simulink library "MBDS_Subsystems"  (R2018b)
settings: Solver=ode45  StartTime=0.0  StopTime=10.0  RelTol=1e-3
libraries: KIBES_Signal x1429, MBDS_Modules x44, simulink x2
(part 10 of 15)

== system MBDS_Subsystems/SUB_IoControl/AnalogsSupply ==
  bo_SendEnable : Inport
  AND : Subsystem  InitFcn=|  mask(AND){MBDS_LibraryBlock=on, BitwiseMode=off, Inputs=2, UseBitMask=off, BitMask='A7', OutDataTypeStr=Inherit: Inherit via back propagation, MBDS_BlockVersion=08.20.02}
      | if(exist('MBDS_BlockCallback', 'file'))
      |    MBDS_BlockCallback('Update', gcb);
      | end
      mask prompts: MBDS_LibraryBlock "MBDS library block"; BitwiseMode "Use 'bitwise' mode"; Inputs "Number of input ports:"; UseBitMask "Use bit mask"; BitMask "Bit mask:"; OutDataTypeStr "Output data type:"; MBDS_BlockVersion "Version:"
      mask help: Logical or bitwise AND operator. For multiple inputs, operators are applied across the inputs. For a single input, operators are applied across the input vector. In bitwise mode a bit mask can be applied onto single input signals.
      mask init: same as MBDS_Subsystems/SUB_DateTime/AND
      mask Help: eval(['open([workdir(''library_dir:''),''\Blockset\help\'',get_param(gcb,''MaskType''),''.html''])'])
      mask Callback BitwiseMode:
      | if(exist('MBDS_BlockCallback', 'file'))
      |    MBDS_BlockCallback('BitwiseMode', gcb);
      | end
      mask Callback Inputs:
      | if(exist('MBDS_BlockCallback', 'file'))
      |    MBDS_BlockCallback('Inputs', gcb);
      | end
      mask Callback UseBitMask:
      | if(exist('MBDS_BlockCallback', 'file'))
      |    MBDS_BlockCallback('UseBitMask', gcb);
      | end
      mask Callback BitMask:
      | if(exist('MBDS_BlockCallback', 'file'))
      |    MBDS_BlockCallback('BitMask', gcb);
      | end
      mask TypeOptions OutDataTypeStr: Inherit: Inherit via back propagation | int8 | uint8 | int16 | uint16 | int32 | uint32 | boolean
      mask Callback OutDataTypeStr:
      | % Adopt Value
      | if(exist('MBDS_BlockCallback', 'file'))
      |    MBDS_BlockCallback('OutDataTypeStr', gcb);
      | end
      mask DialogControl ParameterTabVar0 Prompt: Main
      mask DialogControl ParameterTabVar01 Prompt: Signal Attributes
      mask DialogControl ParameterTabVar012 Prompt: Version
      mask Display:
      | % Show icon or block text
      | if(UseBitMask)
      |    if(isnumeric(BitMask))
      |       BitMaskString = ['0x',dec2hex(floor(BitMask))];
      |    elseif(ischar(BitMask))
      |       BitMaskString = ['0x',upper(BitMask)];
      |    else
      |       BitMaskString = '???';
      |    end
      |    disp(sprintf(['AND\n', BitMaskString]))
      | else
      |    disp('AND')
      | end
  AND1 : Subsystem  InitFcn=|  mask(AND){MBDS_LibraryBlock=on, BitwiseMode=off, Inputs=2, UseBitMask=off, BitMask='A7', OutDataTypeStr=Inherit: Inherit via back propagation, MBDS_BlockVersion=08.20.02}
      | if(exist('MBDS_BlockCallback', 'file'))
      |    MBDS_BlockCallback('Update', gcb);
      | end
      mask prompts: MBDS_LibraryBlock "MBDS library block"; BitwiseMode "Use 'bitwise' mode"; Inputs "Number of input ports:"; UseBitMask "Use bit mask"; BitMask "Bit mask:"; OutDataTypeStr "Output data type:"; MBDS_BlockVersion "Version:"
      mask help: Logical or bitwise AND operator. For multiple inputs, operators are applied across the inputs. For a single input, operators are applied across the input vector. In bitwise mode a bit mask can be applied onto single input signals.
      mask init: same as MBDS_Subsystems/SUB_DateTime/AND
      mask Help: eval(['open([workdir(''library_dir:''),''\Blockset\help\'',get_param(gcb,''MaskType''),''.html''])'])
      mask Callback BitwiseMode:
      | if(exist('MBDS_BlockCallback', 'file'))
      |    MBDS_BlockCallback('BitwiseMode', gcb);
      | end
      mask Callback Inputs:
      | if(exist('MBDS_BlockCallback', 'file'))
      |    MBDS_BlockCallback('Inputs', gcb);
      | end
      mask Callback UseBitMask:
      | if(exist('MBDS_BlockCallback', 'file'))
      |    MBDS_BlockCallback('UseBitMask', gcb);
      | end
      mask Callback BitMask:
      | if(exist('MBDS_BlockCallback', 'file'))
      |    MBDS_BlockCallback('BitMask', gcb);
      | end
      mask TypeOptions OutDataTypeStr: Inherit: Inherit via back propagation | int8 | uint8 | int16 | uint16 | int32 | uint32 | boolean
      mask Callback OutDataTypeStr:
      | % Adopt Value
      | if(exist('MBDS_BlockCallback', 'file'))
      |    MBDS_BlockCallback('OutDataTypeStr', gcb);
      | end
      mask DialogControl ParameterTabVar0 Prompt: Main
      mask DialogControl ParameterTabVar01 Prompt: Signal Attributes
      mask DialogControl ParameterTabVar012 Prompt: Version
      mask Display:
      | % Show icon or block text
      | if(UseBitMask)
      |    if(isnumeric(BitMask))
      |       BitMaskString = ['0x',dec2hex(floor(BitMask))];
      |    elseif(ischar(BitMask))
      |       BitMaskString = ['0x',upper(BitMask)];
      |    else
      |       BitMaskString = '???';
      |    end
      |    disp(sprintf(['AND\n', BitMaskString]))
      | else
      |    disp('AND')
      | end
  AND2 : Subsystem  InitFcn=|  mask(AND){MBDS_LibraryBlock=on, BitwiseMode=off, Inputs=2, UseBitMask=off, BitMask='A7', OutDataTypeStr=Inherit: Inherit via back propagation, MBDS_BlockVersion=08.20.02}
      | if(exist('MBDS_BlockCallback', 'file'))
      |    MBDS_BlockCallback('Update', gcb);
      | end
      mask prompts: MBDS_LibraryBlock "MBDS library block"; BitwiseMode "Use 'bitwise' mode"; Inputs "Number of input ports:"; UseBitMask "Use bit mask"; BitMask "Bit mask:"; OutDataTypeStr "Output data type:"; MBDS_BlockVersion "Version:"
      mask help: Logical or bitwise AND operator. For multiple inputs, operators are applied across the inputs. For a single input, operators are applied across the input vector. In bitwise mode a bit mask can be applied onto single input signals.
      mask init: same as MBDS_Subsystems/SUB_DateTime/AND
      mask Help: eval(['open([workdir(''library_dir:''),''\Blockset\help\'',get_param(gcb,''MaskType''),''.html''])'])
      mask Callback BitwiseMode:
      | if(exist('MBDS_BlockCallback', 'file'))
      |    MBDS_BlockCallback('BitwiseMode', gcb);
      | end
      mask Callback Inputs:
      | if(exist('MBDS_BlockCallback', 'file'))
      |    MBDS_BlockCallback('Inputs', gcb);
      | end
      mask Callback UseBitMask:
      | if(exist('MBDS_BlockCallback', 'file'))
      |    MBDS_BlockCallback('UseBitMask', gcb);
      | end
      mask Callback BitMask:
      | if(exist('MBDS_BlockCallback', 'file'))
      |    MBDS_BlockCallback('BitMask', gcb);
      | end
      mask TypeOptions OutDataTypeStr: Inherit: Inherit via back propagation | int8 | uint8 | int16 | uint16 | int32 | uint32 | boolean
      mask Callback OutDataTypeStr:
      | % Adopt Value
      | if(exist('MBDS_BlockCallback', 'file'))
      |    MBDS_BlockCallback('OutDataTypeStr', gcb);
      | end
      mask DialogControl ParameterTabVar0 Prompt: Main
      mask DialogControl ParameterTabVar01 Prompt: Signal Attributes
      mask DialogControl ParameterTabVar012 Prompt: Version
      mask Display:
      | % Show icon or block text
      | if(UseBitMask)
      |    if(isnumeric(BitMask))
      |       BitMaskString = ['0x',dec2hex(floor(BitMask))];
      |    elseif(ischar(BitMask))
      |       BitMaskString = ['0x',upper(BitMask)];
      |    else
      |       BitMaskString = '???';
      |    end
      |    disp(sprintf(['AND\n', BitMaskString]))
      | else
      |    disp('AND')
      | end
  Constant1 : Constant  InitFcn=|  Value=0  OutDataTypeStr=uint16
      | if(exist('MBDS_BlockCallback', 'file'))
      |    MBDS_BlockCallback('Update', gcb);  
      | end
  EQ : Subsystem  InitFcn=|  mask(EQ){MBDS_LibraryBlock=on, InputSameDT=on, MBDS_BlockVersion=08.20.02}
      | if(exist('MBDS_BlockCallback', 'file'))
      |    MBDS_BlockCallback('Update', gcb);
      | end
      mask prompts: MBDS_LibraryBlock "MBDS library block"; InputSameDT "Require all inputs to have the same data type"; MBDS_BlockVersion "Block version:"
      mask help: The block compares if both input signals are equal.
      mask init: same as MBDS_Subsystems/SUB_DateTime/AND
      mask Help: eval(['open([workdir(''library_dir:''),''\Blockset\help\'',get_param(gcb,''MaskType''),''.html''])'])
      mask Callback InputSameDT:
      | % Adopt value
      | if(exist('MBDS_BlockCallback', 'file'))
      |    MBDS_BlockCallback('InputSameDT', gcb);
      | end
      mask DialogControl ParameterTabVar0 Prompt: Signal Attributes
      mask DialogControl ParameterTabVar01 Prompt: Version
      mask Display:
      | % Show icon or block text
      | if(exist('MBDS_BlockCallback', 'file'))
      |    image(imread('EQ.tif','tif'),[0.35,0.35,0.355,0.25])
      |    disp('')
      | else
      |    disp(sprintf('=='));
      | end
  in_DIAG_AnalogSupply.OUT_ANA_PWR_01_DIAG : KIBES_Signal/KIBES_Signal  MBDS_LibraryBlock=on  DatabaseKey=745  SignalName=DIAG_AnalogSupply.OUT_ANA_PWR_01_DIAG  SymbolName=DIAG_AnalogSupply_OUT_ANA_PWR_01_DIAG_000745  DataType=uint16  Init=1  Slope=1  Bias=0  DataSize=1  fpDataType=uint16  BlockIOType=Inport  DeviceType=0
  in_DIAG_AnalogSupply.OUT_ANA_PWR_02_DIAG : KIBES_Signal/KIBES_Signal  MBDS_LibraryBlock=on  DatabaseKey=747  SignalName=DIAG_AnalogSupply.OUT_ANA_PWR_02_DIAG  SymbolName=DIAG_AnalogSupply_OUT_ANA_PWR_02_DIAG_000747  DataType=uint16  Init=1  Slope=1  Bias=0  DataSize=1  fpDataType=uint16  BlockIOType=Inport  DeviceType=0
  in_DIAG_AnalogSupply.OUT_ANA_PWR_03_DIAG : KIBES_Signal/KIBES_Signal  MBDS_LibraryBlock=on  DatabaseKey=749  SignalName=DIAG_AnalogSupply.OUT_ANA_PWR_03_DIAG  SymbolName=DIAG_AnalogSupply_OUT_ANA_PWR_03_DIAG_000749  DataType=uint16  Init=1  Slope=1  Bias=0  DataSize=1  fpDataType=uint16  BlockIOType=Inport  DeviceType=0
  in_IN_AnalogSupply.OUT_ANA_PWR_01 : KIBES_Signal/KIBES_Signal  MBDS_LibraryBlock=on  DatabaseKey=744  SignalName=IN_AnalogSupply.OUT_ANA_PWR_01  SymbolName=IN_AnalogSupply_OUT_ANA_PWR_01_000744  DataType=uint16  Init=0  Slope=1  Bias=0  DataSize=1  fpDataType=uint16  BlockIOType=Inport  DeviceType=0
  in_IN_AnalogSupply.OUT_ANA_PWR_02 : KIBES_Signal/KIBES_Signal  MBDS_LibraryBlock=on  DatabaseKey=746  SignalName=IN_AnalogSupply.OUT_ANA_PWR_02  SymbolName=IN_AnalogSupply_OUT_ANA_PWR_02_000746  DataType=uint16  Init=0  Slope=1  Bias=0  DataSize=1  fpDataType=uint16  BlockIOType=Inport  DeviceType=0
  in_IN_AnalogSupply.OUT_ANA_PWR_03 : KIBES_Signal/KIBES_Signal  MBDS_LibraryBlock=on  DatabaseKey=748  SignalName=IN_AnalogSupply.OUT_ANA_PWR_03  SymbolName=IN_AnalogSupply_OUT_ANA_PWR_03_000748  DataType=uint16  Init=0  Slope=1  Bias=0  DataSize=1  fpDataType=uint16  BlockIOType=Inport  DeviceType=0
  in_IN_PCAN.Rx_Ctrl.Out_Ctrl.MessageState : KIBES_Signal/KIBES_Signal  MBDS_LibraryBlock=on  DatabaseKey=1715  SignalName=IN_PCAN.Rx_Ctrl.Out_Ctrl.MessageState  SymbolName=IN_PCAN_Rx_Ctrl_Out_Ctrl_MessageState_001715  DataType=uint16  Init=0  Slope=1  Bias=0  DataSize=1  fpDataType=uint16  BlockIOType=Inport  DeviceType=0
  in_IN_PCAN.Rx_Ctrl.Out_Ctrl.Out_Supply_ANA_01_Ctrl : KIBES_Signal/KIBES_Signal  MBDS_LibraryBlock=on  DatabaseKey=1684  SignalName=IN_PCAN.Rx_Ctrl.Out_Ctrl.Out_Supply_ANA_01_Ctrl  SymbolName=IN_PCAN_Rx_Ctrl_Out_Ctrl_Out_Supply_ANA_01_Ctrl_001684  DataType=boolean  Init=0  Slope=1  Bias=0  DataSize=1  fpDataType=boolean  BlockIOType=Inport  DeviceType=0
  in_IN_PCAN.Rx_Ctrl.Out_Ctrl.Out_Supply_ANA_02_Ctrl : KIBES_Signal/KIBES_Signal  MBDS_LibraryBlock=on  DatabaseKey=1683  SignalName=IN_PCAN.Rx_Ctrl.Out_Ctrl.Out_Supply_ANA_02_Ctrl  SymbolName=IN_PCAN_Rx_Ctrl_Out_Ctrl_Out_Supply_ANA_02_Ctrl_001683  DataType=boolean  Init=0  Slope=1  Bias=0  DataSize=1  fpDataType=boolean  BlockIOType=Inport  DeviceType=0
  in_IN_PCAN.Rx_Ctrl.Out_Ctrl.Out_Supply_ANA_03_Ctrl : KIBES_Signal/KIBES_Signal  MBDS_LibraryBlock=on  DatabaseKey=1682  SignalName=IN_PCAN.Rx_Ctrl.Out_Ctrl.Out_Supply_ANA_03_Ctrl  SymbolName=IN_PCAN_Rx_Ctrl_Out_Ctrl_Out_Supply_ANA_03_Ctrl_001682  DataType=boolean  Init=0  Slope=1  Bias=0  DataSize=1  fpDataType=boolean  BlockIOType=Inport  DeviceType=0
  out_OUT_DigitalOutputsSTATIC.OUT_SUP_ANA_01 : KIBES_Signal/KIBES_Signal  MBDS_LibraryBlock=on  DatabaseKey=340  SignalName=OUT_DigitalOutputsSTATIC.OUT_SUP_ANA_01  SymbolName=OUT_DigitalOutputsSTATIC_OUT_SUP_ANA_01_000340  DataType=boolean  Init=0  Slope=1  Bias=0  DataSize=1  fpDataType=boolean  BlockIOType=Outport  DeviceType=0
  out_OUT_DigitalOutputsSTATIC.OUT_SUP_ANA_02 : KIBES_Signal/KIBES_Signal  MBDS_LibraryBlock=on  DatabaseKey=341  SignalName=OUT_DigitalOutputsSTATIC.OUT_SUP_ANA_02  SymbolName=OUT_DigitalOutputsSTATIC_OUT_SUP_ANA_02_000341  DataType=boolean  Init=0  Slope=1  Bias=0  DataSize=1  fpDataType=boolean  BlockIOType=Outport  DeviceType=0
  out_OUT_DigitalOutputsSTATIC.OUT_SUP_ANA_03 : KIBES_Signal/KIBES_Signal  MBDS_LibraryBlock=on  DatabaseKey=342  SignalName=OUT_DigitalOutputsSTATIC.OUT_SUP_ANA_03  SymbolName=OUT_DigitalOutputsSTATIC_OUT_SUP_ANA_03_000342  DataType=boolean  Init=0  Slope=1  Bias=0  DataSize=1  fpDataType=boolean  BlockIOType=Outport  DeviceType=0
  out_OUT_PCAN.Tx_Pwr.Out_Supply_ANA_01_Sts.MessageEnable : KIBES_Signal/KIBES_Signal  MBDS_LibraryBlock=on  DatabaseKey=1790  SignalName=OUT_PCAN.Tx_Pwr.Out_Supply_ANA_01_Sts.MessageEnable  SymbolName=OUT_PCAN_Tx_Pwr_Out_Supply_ANA_01_Sts_MessageEnable_001790  DataType=boolean  Init=0  Slope=1  Bias=0  DataSize=1  fpDataType=boolean  BlockIOType=Outport  DeviceType=0
  out_OUT_PCAN.Tx_Pwr.Out_Supply_ANA_01_Sts.Supply_ANA_DIAG : KIBES_Signal/KIBES_Signal  MBDS_LibraryBlock=on  DatabaseKey=1784  SignalName=OUT_PCAN.Tx_Pwr.Out_Supply_ANA_01_Sts.Supply_ANA_DIAG  SymbolName=OUT_PCAN_Tx_Pwr_Out_Supply_ANA_01_Sts_Supply_ANA_DIAG_001784  DataType=uint16  Init=0  Slope=1  Bias=0  DataSize=1  fpDataType=uint16  BlockIOType=Outport  DeviceType=0
  out_OUT_PCAN.Tx_Pwr.Out_Supply_ANA_01_Sts.Supply_ANA_Val : KIBES_Signal/KIBES_Signal  MBDS_LibraryBlock=on  DatabaseKey=1785  SignalName=OUT_PCAN.Tx_Pwr.Out_Supply_ANA_01_Sts.Supply_ANA_Val  SymbolName=OUT_PCAN_Tx_Pwr_Out_Supply_ANA_01_Sts_Supply_ANA_Val_001785  DataType=uint16  Init=0  Slope=1  Bias=0  DataSize=1  fpDataType=uint16  BlockIOType=Outport  DeviceType=0
  out_OUT_PCAN.Tx_Pwr.Out_Supply_ANA_02_Sts.MessageEnable : KIBES_Signal/KIBES_Signal  MBDS_LibraryBlock=on  DatabaseKey=1791  SignalName=OUT_PCAN.Tx_Pwr.Out_Supply_ANA_02_Sts.MessageEnable  SymbolName=OUT_PCAN_Tx_Pwr_Out_Supply_ANA_02_Sts_MessageEnable_001791  DataType=boolean  Init=0  Slope=1  Bias=0  DataSize=1  fpDataType=boolean  BlockIOType=Outport  DeviceType=0
  out_OUT_PCAN.Tx_Pwr.Out_Supply_ANA_02_Sts.Supply_ANA_DIAG : KIBES_Signal/KIBES_Signal  MBDS_LibraryBlock=on  DatabaseKey=1786  SignalName=OUT_PCAN.Tx_Pwr.Out_Supply_ANA_02_Sts.Supply_ANA_DIAG  SymbolName=OUT_PCAN_Tx_Pwr_Out_Supply_ANA_02_Sts_Supply_ANA_DIAG_001786  DataType=uint16  Init=0  Slope=1  Bias=0  DataSize=1  fpDataType=uint16  BlockIOType=Outport  DeviceType=0
  out_OUT_PCAN.Tx_Pwr.Out_Supply_ANA_02_Sts.Supply_ANA_Val : KIBES_Signal/KIBES_Signal  MBDS_LibraryBlock=on  DatabaseKey=1787  SignalName=OUT_PCAN.Tx_Pwr.Out_Supply_ANA_02_Sts.Supply_ANA_Val  SymbolName=OUT_PCAN_Tx_Pwr_Out_Supply_ANA_02_Sts_Supply_ANA_Val_001787  DataType=uint16  Init=0  Slope=1  Bias=0  DataSize=1  fpDataType=uint16  BlockIOType=Outport  DeviceType=0
  out_OUT_PCAN.Tx_Pwr.Out_Supply_ANA_03_Sts.MessageEnable : KIBES_Signal/KIBES_Signal  MBDS_LibraryBlock=on  DatabaseKey=1792  SignalName=OUT_PCAN.Tx_Pwr.Out_Supply_ANA_03_Sts.MessageEnable  SymbolName=OUT_PCAN_Tx_Pwr_Out_Supply_ANA_03_Sts_MessageEnable_001792  DataType=boolean  Init=0  Slope=1  Bias=0  DataSize=1  fpDataType=boolean  BlockIOType=Outport  DeviceType=0
  out_OUT_PCAN.Tx_Pwr.Out_Supply_ANA_03_Sts.Supply_ANA_DIAG : KIBES_Signal/KIBES_Signal  MBDS_LibraryBlock=on  DatabaseKey=1788  SignalName=OUT_PCAN.Tx_Pwr.Out_Supply_ANA_03_Sts.Supply_ANA_DIAG  SymbolName=OUT_PCAN_Tx_Pwr_Out_Supply_ANA_03_Sts_Supply_ANA_DIAG_001788  DataType=uint16  Init=0  Slope=1  Bias=0  DataSize=1  fpDataType=uint16  BlockIOType=Outport  DeviceType=0
  out_OUT_PCAN.Tx_Pwr.Out_Supply_ANA_03_Sts.Supply_ANA_Val : KIBES_Signal/KIBES_Signal  MBDS_LibraryBlock=on  DatabaseKey=1789  SignalName=OUT_PCAN.Tx_Pwr.Out_Supply_ANA_03_Sts.Supply_ANA_Val  SymbolName=OUT_PCAN_Tx_Pwr_Out_Supply_ANA_03_Sts_Supply_ANA_Val_001789  DataType=uint16  Init=0  Slope=1  Bias=0  DataSize=1  fpDataType=uint16  BlockIOType=Outport  DeviceType=0
  wires:
  AND2/1(y) -> out_OUT_DigitalOutputsSTATIC.OUT_SUP_ANA_03/1
  AND1/1(y) -> out_OUT_DigitalOutputsSTATIC.OUT_SUP_ANA_02/1
  in_IN_PCAN.Rx_Ctrl.Out_Ctrl.Out_Supply_ANA_03_Ctrl/1 -> AND2/2(u2)
  in_IN_PCAN.Rx_Ctrl.Out_Ctrl.Out_Supply_ANA_02_Ctrl/1 -> AND1/2(u2)
  AND/1(y) -> out_OUT_DigitalOutputsSTATIC.OUT_SUP_ANA_01/1
  in_IN_PCAN.Rx_Ctrl.Out_Ctrl.Out_Supply_ANA_01_Ctrl/1 -> AND/2(u2)
  [boCtrlValid] -> AND/1(u1), AND1/1(u1), AND2/1(u1)
  EQ/1(y) -> [boCtrlValid]
  in_IN_PCAN.Rx_Ctrl.Out_Ctrl.MessageState/1 -> EQ/1(u1)
  Constant1/1 -> EQ/2(u2)
  in_IN_AnalogSupply.OUT_ANA_PWR_03/1 -> out_OUT_PCAN.Tx_Pwr.Out_Supply_ANA_03_Sts.Supply_ANA_Val/1
  in_IN_AnalogSupply.OUT_ANA_PWR_02/1 -> out_OUT_PCAN.Tx_Pwr.Out_Supply_ANA_02_Sts.Supply_ANA_Val/1
  in_IN_AnalogSupply.OUT_ANA_PWR_01/1 -> out_OUT_PCAN.Tx_Pwr.Out_Supply_ANA_01_Sts.Supply_ANA_Val/1
  bo_SendEnable/1 -> out_OUT_PCAN.Tx_Pwr.Out_Supply_ANA_02_Sts.MessageEnable/1, out_OUT_PCAN.Tx_Pwr.Out_Supply_ANA_03_Sts.MessageEnable/1, out_OUT_PCAN.Tx_Pwr.Out_Supply_ANA_01_Sts.MessageEnable/1
  in_DIAG_AnalogSupply.OUT_ANA_PWR_01_DIAG/1 -> out_OUT_PCAN.Tx_Pwr.Out_Supply_ANA_01_Sts.Supply_ANA_DIAG/1
  in_DIAG_AnalogSupply.OUT_ANA_PWR_03_DIAG/1 -> out_OUT_PCAN.Tx_Pwr.Out_Supply_ANA_03_Sts.Supply_ANA_DIAG/1
  in_DIAG_AnalogSupply.OUT_ANA_PWR_02_DIAG/1 -> out_OUT_PCAN.Tx_Pwr.Out_Supply_ANA_02_Sts.Supply_ANA_DIAG/1
